simulink model "Pouziti_Mux_VC_BUS"  (R2020b)
settings: Solver=VariableStepAuto  StartTime=0.0  StopTime=10.0  RelTol=1e-3
settings Model: Creator=jirkovsky  LastModifiedBy=jirkovsky

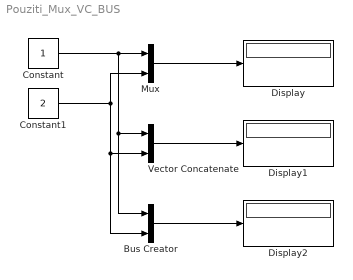
== system Pouziti_Mux_VC_BUS ==
  Bus Creator : BusCreator  Inputs=2
  Constant : Constant
  Constant1 : Constant  Value=2
  Display : Display
  Display1 : Display
  Display2 : Display
  Mux : Mux  Inputs=2
  Vector Concatenate : Concatenate
  wires:
  Constant/1 -> Vector Concatenate/1, Bus Creator/1, Mux/1
  Constant1/1 -> Bus Creator/2, Vector Concatenate/2, Mux/2
  Mux/1 -> Display/1
  Vector Concatenate/1 -> Display1/1
  Bus Creator/1 -> Display2/1
